simulink model "mass_spring_damper"  (R2020b)
settings: Solver=ode4  StartTime=0.0  StopTime=10.0  FixedStep=sim_step  RelTol=1e-3  EnableMultiTasking=on
values from neighbouring files (symbols this model uses):
  k = 1    [msd_script.m]
  lambda = lambda_set(i)    [msd_script.m]
  m = m_set(j)    [msd_script.m]
settings Model: Creator=c109799  LastModifiedBy=gonza
settings DataIOCC: ExternalInput=[t', u']  LimitDataPoints=on  LoadExternalInput=on  SaveFormat=Array  ReturnWorkspaceOutputs=off
settings OptimizationCC: ExpressionDepthLimit=2147483647  LifeSpan=inf
settings DebuggingCC: UnderspecifiedInitializationDetection=Classic  MergeDetectMultiDrivingBlocksExec=none  SolverPrmCheckMsg=warning  StateNameClashWarn=warning  SFUnexpectedBacktrackingDiag=warning  SFNoUnconditionalDefaultTransitionDiag=warning  SFExecutionAtInitializationDiag=none  ArithmeticOperatorsInVariantConditions=warning
settings HardwareCC: ProdBitPerPointer=32  ProdBitPerSizeT=32  ProdBitPerPtrDiffT=32  ProdLargestAtomicFloat=None  ProdIntDivRoundTo=Undefined  ProdEndianess=Unspecified  ProdWordSize=32  ProdHWDeviceType=32-bit Generic
settings ModelReferenceCC: PropagateSignalLabelsOutOfModel=off
settings SFSimCC: SimUseLocalCustomCode=off  CustomCodeUndefinedFunction=UseInterfaceOnly
settings RTWCC: RTWUseLocalCustomCode=off
settings CodeAppCC: StateflowObjectComments=on
settings GRTTargetCC: TargetLangStandard=C89/C90 (ANSI)
settings ConfigComp: CovMetricSettings=dw  CovSaveCumulativeToWorkspaceVar=on  CovSaveSingleToWorkspaceVar=on  CovExternalEMLEnable=off

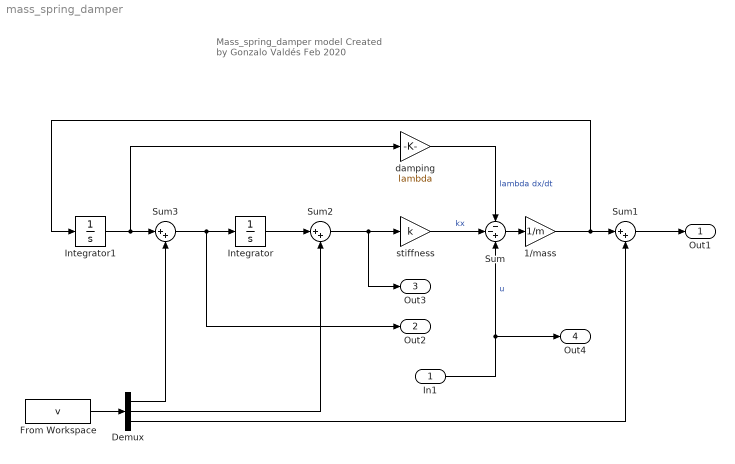
== system mass_spring_damper ==
  note: Mass_spring_damper model
      | Created by Gonzalo Valdés
      | Feb 2020
  In1 : Inport
  1/mass : Gain  Gain=1/m
  Demux : Demux  Outputs=3
  From Workspace : FromWorkspace  VariableName=v
  Integrator : Integrator  ContinuousStateAttributes='x'
  Integrator1 : Integrator  ContinuousStateAttributes='dx'
  Sum : Sum  Inputs=--+
  Sum1 : Sum  Inputs=|++
  Sum2 : Sum  Inputs=|++
  Sum3 : Sum  Inputs=|++
  damping : Gain  Gain=lambda
  stiffness : Gain  Gain=k
  Out1 : Outport
  Out2 : Outport  Port=2
  Out3 : Outport  Port=3
  Out4 : Outport  Port=4
  wires:
  Integrator1/1 -> Sum3/1, damping/1
  stiffness/1 -> Sum/2  "kx"
  damping/1 -> Sum/1  "lambda dx/dt"
  Sum/1 -> 1/mass/1
  1/mass/1 -> Sum1/1, Integrator1/1
  Sum1/1 -> Out1/1
  In1/1 -> Out4/1, Sum/3  "u"
  Integrator/1 -> Sum2/1
  Sum3/1 -> Out2/1, Integrator/1
  From Workspace/1 -> Demux/1
  Demux/1 -> Sum3/2
  Demux/2 -> Sum2/2
  Demux/3 -> Sum1/2
  Sum2/1 -> Out3/1, stiffness/1
